simulink model "simpleDemo"  (R2024a)
settings: Solver=FixedStepAuto  StartTime=0.0  StopTime=1  RelTol=1e-3
model workspace (MAT data in the model file):
  SL_ROS_VariableLengthArrays_MaxSizes.CommonInfo.ArrayTruncateAction = 'EmitWarning'
  SL_ROS_VariableLengthArrays_MaxSizes.MsgTypeMap = containers.Map
  SL_ROS_VariableLengthArrays_MaxSizes.MsgTypeMap.serialization.keys = {'std_msgs/Int8MultiArray'}
  SL_ROS_VariableLengthArrays_MaxSizes.MsgTypeMap.serialization.values{1}.PropertyName = 'data'
  SL_ROS_VariableLengthArrays_MaxSizes.MsgTypeMap.serialization.values{1}.DataType = 'int8'
  SL_ROS_VariableLengthArrays_MaxSizes.MsgTypeMap.serialization.values{1}.MaxLength = 10000
  SL_ROS_VariableLengthArrays_MaxSizes.MsgTypeMap.serialization.uniformity = 0
  SL_ROS_VariableLengthArrays_MaxSizes.MsgTypeMap.serialization.keyType = 'char'
  SL_ROS_VariableLengthArrays_MaxSizes.MsgTypeMap.serialization.valueType = 'any'
libraries: roshelperlib x4
settings Model: DataDictionary=ros2lib.sldd  Creator=cstabile  LastModifiedBy=cstabile
settings OptimizationCC: EnhancedBackFolding=on  PassReuseOutputArgsAs=Individual arguments  ZeroExternalMemoryAtStartup=off  ZeroInternalMemoryAtStartup=off  MaxStackSize=64  OptimizeBlockOrder=speed  DifferentSizesBufferReuse=on  OptimizationCustomize=off  EfficientTunableParamExpr=on
settings DebuggingCC: ParameterTunabilityLossMsg=error
settings SFSimCC: MATLABDynamicMemAlloc=off
settings RTWCC: Description=Embedded Coder  SystemTargetFile=ert.tlc  HardwareBoard=Robot Operating System 2 (ROS 2)  TLCOptions="-aInlineSetEventsForThisBaseRateFcn=TLC_FALSE -aSuppressMultiTaskScheduler=TLC_FALSE  -aRateBasedStepFcn=0"  TemplateMakefile=ert_default_tmf  Toolchain=Colcon Tools  TargetLang=C++
settings CodeAppCC: ForceParamTrailComments=on  IgnoreCustomStorageClasses=off  OperatorAnnotations=on  SimulinkDataObjDesc=on  SFDataObjDesc=on  InsertBlockDesc=on
settings ERTTargetCC: CodeInterfacePackaging=C++ class  RootIOFormat=Structure reference  SubcomponentRootIOFormat=Individual arguments
settings ConfigComp: CovAccelSimSupport=on

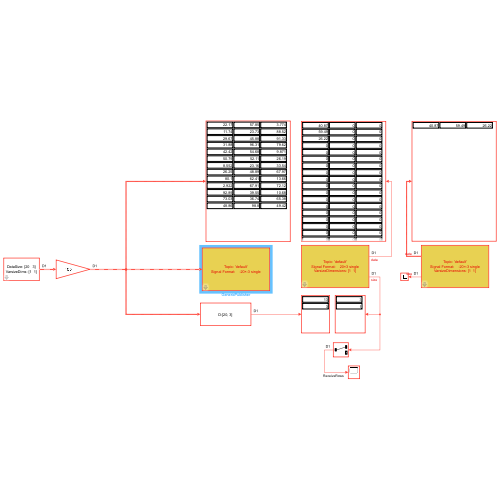
[thumbnail: Simulink's stored preview of the top-level diagram]
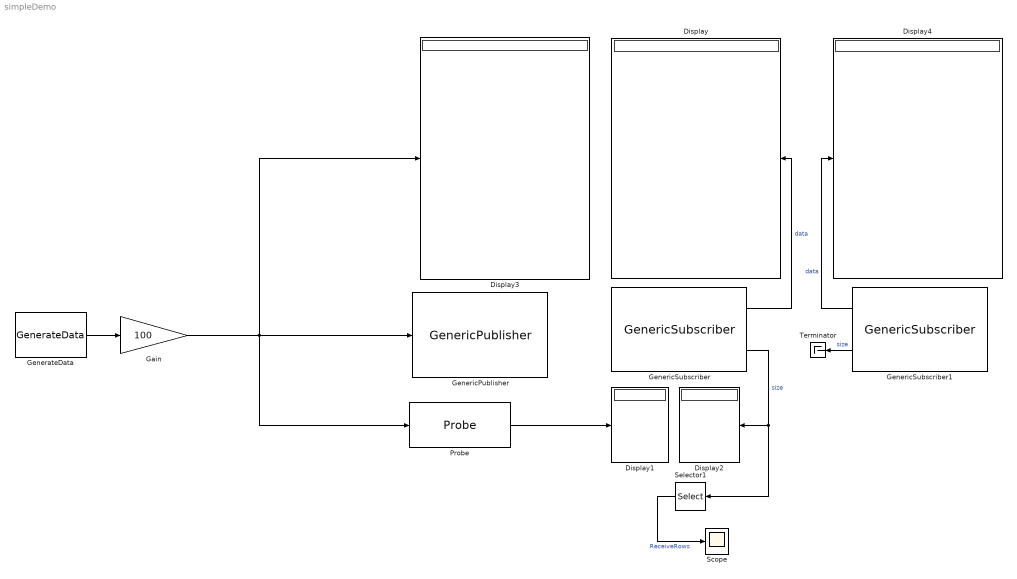
== system simpleDemo ==
  Display{,1..4} (5 alike) : Display
  Gain : Gain  Gain=100
  GenerateData : roshelperlib/GenerateData  dataSize=[20 3]  varsizeDims=[1 1]
  GenericPublisher : roshelperlib/GenericPublisher  userDataType=single  dims=[20 3]  topicName='default'  isVarsize=on  varsizeDims=[1 1]
  GenericSubscriber : roshelperlib/GenericSubscriber  userDataType=single  dims=[20 3]  topicName='default'  isVarsize=on  varsizeDims=[1 1]  returnFixedTF=on
  GenericSubscriber1 : roshelperlib/GenericSubscriber  userDataType=single  dims=[20 3]  topicName='default'  isVarsize=on  varsizeDims=[1 1]  returnFixedTF=off
  Probe : Probe  ProbeWidth=off  ProbeSampleTime=off  ProbeComplexSignal=off  ProbeSignalDimensions=on
  Scope : Scope
  Selector1 : Selector  InputPortWidth=2  IndexOptions=Index vector (dialog)  Indices=1  OutputSizes=1
  Terminator : Terminator
  wires:
  GenerateData/1 -> Gain/1
  GenericSubscriber/1 -> Display/1  "data"
  GenericSubscriber/2 -> Selector1/1, Display2/1  "size"
  Probe/1 -> Display1/1
  Selector1/1 -> Scope/1  "ReceiveRows"
  Gain/1 -> GenericPublisher/1, Probe/1, Display3/1
  GenericSubscriber1/1 -> Display4/1  "data"
  GenericSubscriber1/2 -> Terminator/1  "size"
